simulink model "Project7"  (R2018b)
settings: Solver=VariableStepAuto  StartTime=0.0  StopTime=Sim_Time  RelTol=1e-3
values from neighbouring files (symbols this model uses):
  b = 10    [Project7_run.m]
  k = 20    [Project7_run.m]
  Kd = 50    [Project7_run.m]
  Ki = 300    [Project7_run.m]
  Kp = 350    [Project7_run.m]
  M = 1    [Project7_run.m]
settings Model: Creator=Ismael  LastModifiedBy=Ismael

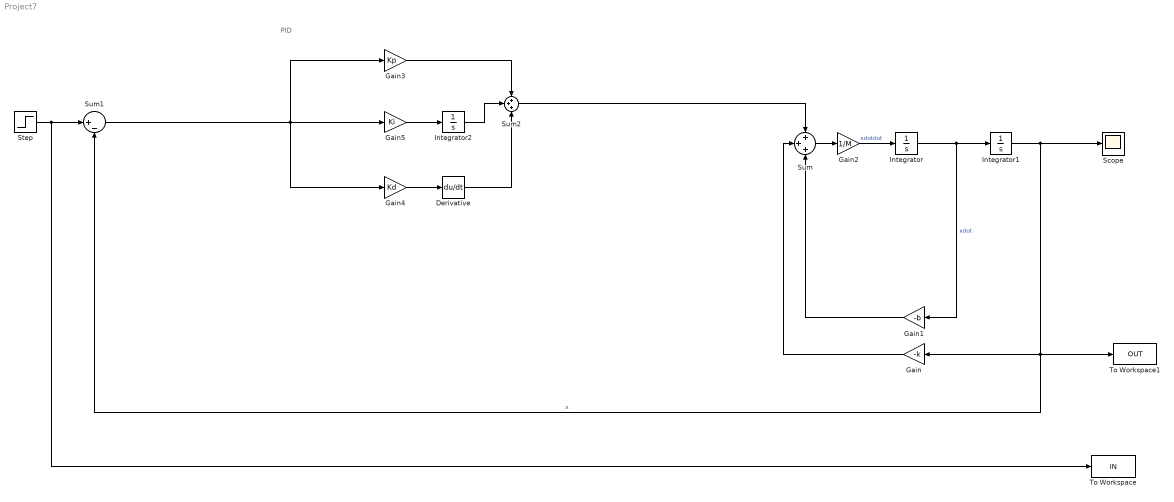
== system Project7 ==
  note: PID
  Derivative : Derivative
  Gain : Gain  Gain=-k
  Gain1 : Gain  Gain=-b
  Gain2 : Gain  Gain=1/M
  Gain3 : Gain  Gain=Kp
  Gain4 : Gain  Gain=Kd
  Gain5 : Gain  Gain=Ki
  Integrator : Integrator
  Integrator1 : Integrator
  Integrator2 : Integrator
  Scope : Scope
  Step : Step  SampleTime=0
  Sum : Sum  Inputs=+++
  Sum1 : Sum  Inputs=|+-
  Sum2 : Sum  Inputs=+++
  To Workspace : ToWorkspace  VariableName=IN  SaveFormat=Timeseries  SampleTime=-1
  To Workspace1 : ToWorkspace  VariableName=OUT  SaveFormat=Timeseries  SampleTime=-1
  wires:
  Sum/1 -> Gain2/1
  Integrator1/1 -> Sum1/2, To Workspace1/1, Gain/1, Scope/1  "x"
  Integrator/1 -> Gain1/1, Integrator1/1  "xdot"
  Gain2/1 -> Integrator/1  "xdotdot"
  Gain/1 -> Sum/2
  Gain1/1 -> Sum/3
  Step/1 -> To Workspace/1, Sum1/1
  Sum2/1 -> Sum/1
  Derivative/1 -> Sum2/3
  Gain5/1 -> Integrator2/1
  Gain4/1 -> Derivative/1
  Sum1/1 -> Gain3/1, Gain5/1, Gain4/1
  Gain3/1 -> Sum2/1
  Integrator2/1 -> Sum2/2
